simulink model "model"  (R2022a)
settings: Solver=VariableStepAuto  StartTime=0.0  StopTime=10.0  RelTol=1e-3
settings Model: Creator=Kirill  LastModifiedBy=Kirill

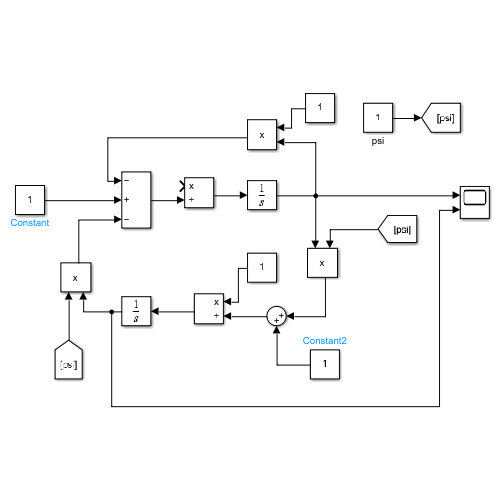
[thumbnail: Simulink's stored preview of the top-level diagram]
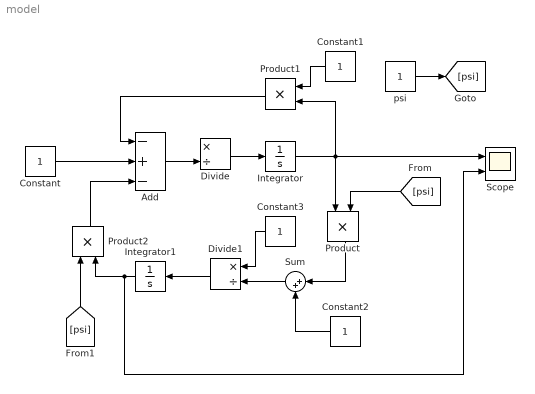
== system model ==
  Add : Sum  Inputs=-+-
  Constant{,1..3} (4 alike) : Constant
  Divide : Product  Inputs=*/
  Divide1 : Product  Inputs=*/
  Integrator : Integrator
  Integrator1 : Integrator
  Product : Product
  Product1 : Product
  Product2 : Product
  Scope : Scope  NumInputPorts=2
  Sum : Sum  Inputs=|++
  psi : Constant
  wires:
  Constant/1 -> Add/2
  Add/1 -> Divide/2
  Divide/1 -> Integrator/1
  Integrator/1 -> Scope/1, Product1/2, Product/1
  Constant1/1 -> Product1/1
  Product1/1 -> Add/1
  psi/1 -> [psi]
  [psi] -> Product/2
  Product/1 -> Sum/1
  Constant2/1 -> Sum/2
  Sum/1 -> Divide1/2
  Constant3/1 -> Divide1/1
  Divide1/1 -> Integrator1/1
  Integrator1/1 -> Scope/2, Product2/2
  [psi] -> Product2/1
  Product2/1 -> Add/3
